simulink model "Modelling_dc_motor"  (R2024a)
settings: Solver=VariableStepAuto  StartTime=0.0  StopTime=10.0  RelTol=1e-3
undefined symbols (not defined in the file): b, J, K, L, R
settings Model: Creator=Admin  LastModifiedBy=Admin

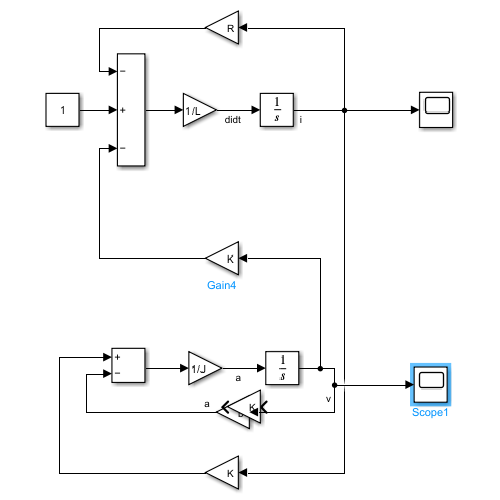
[thumbnail: Simulink's stored preview of the top-level diagram]
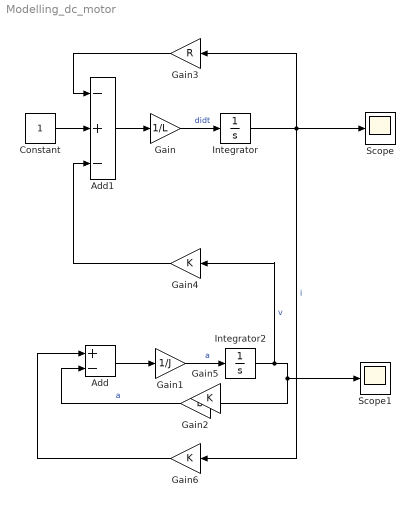
== system Modelling_dc_motor ==
  Add : Sum  Inputs=+-
  Add1 : Sum  Inputs=-+-
  Constant : Constant
  Gain : Gain  Gain=1/L
  Gain1 : Gain  Gain=1/J
  Gain2 : Gain  Gain=b
  Gain3 : Gain  Gain=R
  Gain4 : Gain  Gain=K
  Gain5 : Gain  Gain=K
  Gain6 : Gain  Gain=K
  Integrator : Integrator
  Integrator2 : Integrator
  Scope : Scope
  Scope1 : Scope
  wires:
  Gain/1 -> Integrator/1  "didt"
  Gain1/1 -> Integrator2/1  "a"
  Integrator2/1 -> Gain4/1, Scope1/1, Gain2/1  "v"
  Add/1 -> Gain1/1
  Gain2/1 -> Add/2  "a"
  Integrator/1 -> Gain6/1, Gain3/1, Scope/1  "i"
  Constant/1 -> Add1/2
  Add1/1 -> Gain/1
  Gain3/1 -> Add1/1
  Gain4/1 -> Add1/3
  Gain6/1 -> Add/1
